simulink model "motorai"  (R2018b)
settings: Solver=FixedStepAuto  StartTime=0.0  StopTime=inf  FixedStep=SAMPLE_TIME  RelTol=1e-3
PreLoadFcn:
  | UserSettings
InitFcn:
  | ESTIMATION_SAMPLES = 50;
values from neighbouring files (symbols this model uses):
  ADC_bits = 12    [LQR_control_design.m]    (also in UserSettings.m)
  ADC_Vref = 3.3    [LQR_control_design.m]    (also in UserSettings.m)
  current_gain = 0.5    [LQR_control_design.m]    (also in UserSettings.m)
  current_offset = 1    [LQR_control_design.m]    (also in UserSettings.m)
  DATA_SAMPLING_FREQUENCY = 500    [UserSettings.m]
  K = -K    (= -0.383)    [LQG_control_design.m]    (also in LQR_control_design.m = -(1/R).*B'*Sinf; myLQR.m = -(1/R).*B'*Sinf; myREF.m = [Kw Ki])
  motorParameters = Parameters()    [UserSettings.m]
  omega_gain = 0.5    [LQR_control_design.m]    (also in UserSettings.m)
  omega_offset = 1    [LQR_control_design.m]    (also in UserSettings.m)
  PPR = 1000    [LQR_control_design.m]    (also in UserSettings.m)
  Q = 1/2*inv([(omega_max)^2 0 0; 0 (i_max)^2 0; 0 0 (int_max)^2])    [LQG_control_design.m]    (also in LQR_control_design.m = 1/2*inv([(omega_max)^2 0 ; 0 (i_max)^2]); myLQR.m = 1/2*inv([(omega_max)^2 0; 0 (i_max)^2]))
  R = inv([(v_max)^2])    [LQG_control_design.m]    (also in LQR_control_design.m; myLQR.m)
  SAMPLE_TIME = 5e-5    (= 5e-05)    [UserSettings.m]
  V_ACT = 12    [UserSettings.m]
  Vact = 12    [LQR_control_design.m]
undefined symbols (not defined in the file or in its folder): DiscIntNeverNeededParam
libraries: neural x275, mbedblockslib x7, fl_lib x5, nesl_utility x5, dspswit3 x3, elec_lib x3, powerlib_meascontrol x3, dspbuff3 x2, discretizing x1
(part 1 of 14)
settings Model: Creator=aaronrusso  LastModifiedBy=angel
settings DebuggingCC: LibraryContextMissingDiagnostic=none
settings SFSimCC: SimUseLocalCustomCode=off
settings RTWCC: RTWUseLocalCustomCode=off

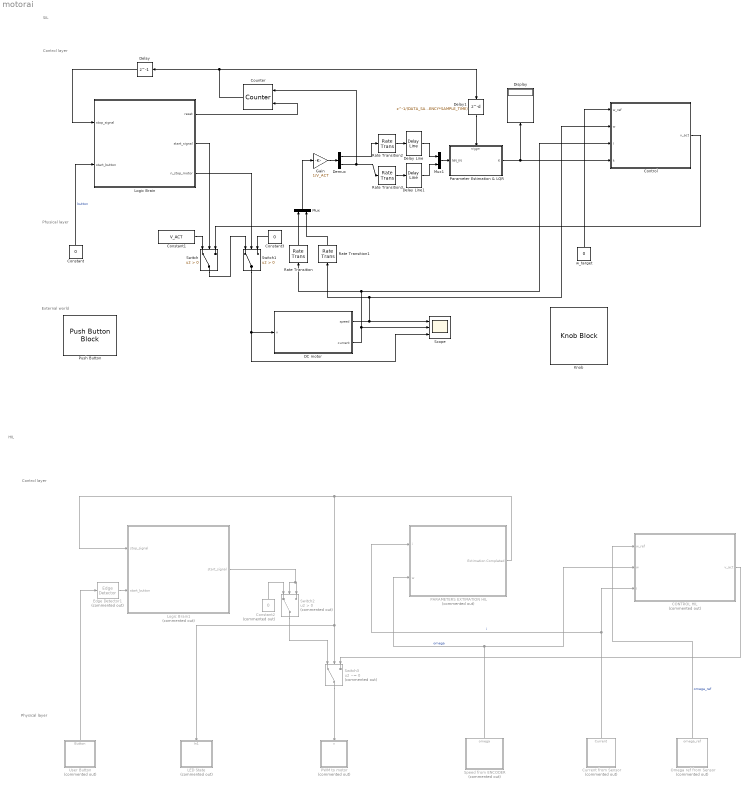
== system motorai ==
  note: HIL
  note: Control layer
  note: Physical layer
  note: External world
  note: Control layer
  note: Physical layer
  note: SIL
  CONTROL HIL : Subsystem  Commented=on
  Constant : Constant  Value=0  SampleTime=SAMPLE_TIME
  Constant1 : Constant  Value=V_ACT  SampleTime=SAMPLE_TIME
  Constant2 : Constant  Commented=on  Value=0
  Constant3 : Constant  Value=0
  "Control " : Subsystem  TreatAsAtomicUnit=on
  Counter : dspswit3/Counter  Direction=Up  CountEvent=Non-zero sample  CounterSize=User defined  MaxCount=(ESTIMATION_SAMPLES)/(DATA_SAMPLING_FREQUENCY*SAMPLE_TIME)  InitialCount=0  Output=Hit  HitValue=(ESTIMATION_SAMPLES)/(DATA_SAMPLING_FREQUENCY*SAMPLE_TIME)  ResetInput=on  SamplesPerFrame=1  Ts=1  CntDtype=double  HitDtype=Logical
  Current from Sensor : Subsystem  Commented=on
      mask Display: image('E:\Università\Magistrale - Advanced Automotive Electronic Engineering\Compliance Design of Automotive Systems\motor-control\MATLAB\images\lowres-INFIN_Icon_Current_02.eps.png');
  DC motor : Subsystem  ClipboardFcn=run('init_throttle.m')
  Delay : Delay  DelayLength=1  InitialCondition=0
  Delay Line : dspbuff3/Delay Line  siz=50  ic=0  directfeed=off  enable_output=off  hold_output=off  OutputFrames=off
      settings: SourceProductName=DSP System Toolbox  SourceProductBaseCode=DS
  Delay Line1 : dspbuff3/Delay Line  siz=50  ic=0  directfeed=off  enable_output=off  hold_output=off  OutputFrames=off
      settings: SourceProductName=DSP System Toolbox  SourceProductBaseCode=DS
  Delay1 : Delay  DelayLength=1/(DATA_SAMPLING_FREQUENCY*SAMPLE_TIME)  InitialCondition=0
  Demux : Demux  Outputs=2
  Display : Display
  Edge Detector1 : powerlib_meascontrol/Logic/Edge Detector  Commented=on  model=Rising  ic=0  Ts=0
      settings: SourceProductName=Simscape Power Systems  SourceProductBaseCode=PS
  Gain : Gain  Gain=1/V_ACT
  Knob : KnobBlock  WebBlockId=276  ScaleMax=500
  LED State : Subsystem  Commented=on
      mask Display: image('E:\Università\Magistrale - Advanced Automotive Electronic Engineering\Compliance Design of Automotive Systems\motor-control\MATLAB\images\led.png');
  Logic Brain : Stateflow chart  TreatAsAtomicUnit=on
  Logic Brain1 : Stateflow chart  Commented=on  TreatAsAtomicUnit=on
  Mux : Mux  Inputs=2
  Mux1 : Mux  Inputs=2
  Omega ref from Sensor : Subsystem  Commented=on
      mask Display: image('E:\Università\Magistrale - Advanced Automotive Electronic Engineering\Compliance Design of Automotive Systems\motor-control\MATLAB\images\65193.png');
  PARAMETERS EXTIMATION HIL : Subsystem  Commented=on
  PWM to motor : Subsystem  Commented=on
      mask Display: image('E:\Università\Magistrale - Advanced Automotive Electronic Engineering\Compliance Design of Automotive Systems\motor-control\MATLAB\images\PWM-Icon.png');
  "Parameter Estimation & LQR " : Subsystem  TreatAsAtomicUnit=on
  Push Button : PushButtonBlock  WebBlockId=163  LabelPosition=Top
  Rate Transition{,1..3} (4 alike) : RateTransition  OutPortSampleTime=1/DATA_SAMPLING_FREQUENCY
  Scope : Scope  NumInputPorts=3
  Speed from ENCODER : Subsystem  Commented=on
      mask Display: image('E:\Università\Magistrale - Advanced Automotive Electronic Engineering\Compliance Design of Automotive Systems\motor-control\MATLAB\images\Cattura.JPG');
  Switch : Switch  Criteria=u2 > Threshold
  Switch1 : Switch  Criteria=u2 > Threshold
  Switch2 : Switch  Commented=on  Criteria=u2 > Threshold
  Switch3 : Switch  Commented=on  Criteria=u2 ~= 0
  User Button : Subsystem  Commented=on
      mask Display: image('E:\Università\Magistrale - Advanced Automotive Electronic Engineering\Compliance Design of Automotive Systems\motor-control\MATLAB\images\red-start-button-5a28dc2fca5281.8598306415126272478287.jpg');
  w_target : Constant  Value=0
  wires:
  Logic Brain1/1(start_signal) -> Switch2/2, Switch2/3
  PARAMETERS EXTIMATION HIL/1(Extimation Completed) -> Logic Brain1/1(stop_signal), LED State/1(In1), Switch3/2
  Constant2/1 -> Switch2/1
  Edge Detector1/1 -> Logic Brain1/2(start_button)
  Current from Sensor/1(Current) -> CONTROL HIL/3(I), PARAMETERS EXTIMATION HIL/1(i)  "i"
  Speed from ENCODER/1(omega) -> CONTROL HIL/2(w), PARAMETERS EXTIMATION HIL/2(w)  "omega"
  Omega ref from Sensor/1(omega_ref) -> CONTROL HIL/1(w_ref)  "omega_ref"
  Switch2/1 -> Switch3/1
  CONTROL HIL/1(v_act) -> Switch3/3
  Switch3/1 -> PWM to motor/1(v)
  User Button/1(Button) -> Edge Detector1/1
  "Parameter Estimation & LQR "/1(K) -> "Control "/4(k), Display/1
  Demux/1 -> Rate Transition2/1
  Counter/1 -> Delay1/1, Delay/1
  Gain/1 -> Demux/1
  Rate Transition2/1 -> Delay Line/1
  Delay/1 -> Logic Brain/1(stop_signal)
  Rate Transition3/1 -> Delay Line1/1
  Rate Transition/1 -> Mux/1
  Rate Transition1/1 -> Mux/2
  Delay Line/1 -> Mux1/1
  Demux/2 -> Rate Transition3/1, Counter/1
  Delay Line1/1 -> Mux1/2
  Delay1/1 -> "Parameter Estimation & LQR "/Trigger
  Mux/1 -> Gain/1
  Mux1/1 -> "Parameter Estimation & LQR "/1(NN_IN)
  Constant/1 -> Logic Brain/2(start_button)  "button"
  Logic Brain/1(reset) -> Counter/2
  Logic Brain/2(start_signal) -> Switch/2
  DC motor/1(speed) -> Scope/1, "Control "/2(w), Rate Transition1/1
  Constant1/1 -> Switch/1
  "Control "/1(v_act) -> Switch/3
  w_target/1 -> "Control "/1(w_ref)
  DC motor/2(current) -> Scope/2, "Control "/3(I), Rate Transition/1
  Logic Brain/3(n_stop_motor) -> Switch1/2
  Switch/1 -> Switch1/1
  Constant3/1 -> Switch1/3
  Switch1/1 -> Scope/3, DC motor/1(v)

== system motorai/CONTROL HIL ==
  w_ref : Inport
  w : Inport  Port=2
  I : Inport  Port=3
  LQR control sim : Subsystem
  Mux1 : Mux  Inputs=2
  v_act : Outport
  wires:
  LQR control sim/1(u) -> v_act/1
  w_ref/1 -> LQR control sim/2(y_ref)
  w/1 -> Mux1/1
  I/1 -> Mux1/2
  Mux1/1 -> LQR control sim/1(x)

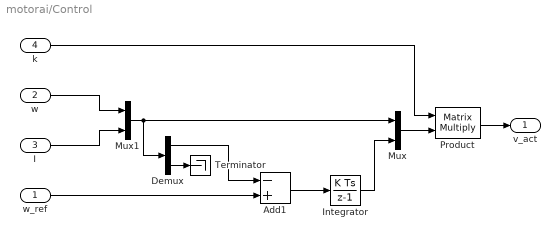
== system motorai/Control  ==
  w_ref : Inport
  w : Inport  Port=2
  I : Inport  Port=3
  k : Inport  Port=4
  Add1 : Sum  Inputs=-+
  Demux : Demux  Outputs=2
  Integrator : DiscreteIntegrator  SampleTime=1.0  ICPrevOutput=DiscIntNeverNeededParam  ICPrevScaledInput=DiscIntNeverNeededParam  mask(DiscretizedDiscreteIntegrator){}
      mask init:
      | %zoh
  Mux : Mux  Inputs=2
  Mux1 : Mux  Inputs=2
  Product : Product  Multiplication=Matrix(*)
  Terminator : Terminator
  v_act : Outport
  wires:
  Integrator/1 -> Mux/2
  Demux/1 -> Add1/1
  I/1 -> Mux1/2
  Product/1 -> v_act/1
  Demux/2 -> Terminator/1
  Add1/1 -> Integrator/1
  w/1 -> Mux1/1
  Mux1/1 -> Mux/1, Demux/1
  w_ref/1 -> Add1/2
  Mux/1 -> Product/2
  k/1 -> Product/1

== system motorai/Current from Sensor ==
  Add : Sum
  Analog Input : mbedblockslib/Analog Input  Pin=PB_0  ReadResultsOnly=off  ConversionTriggerSource=Software  ExternalTriggerType=uint32( 0 )  OutputDataType=double  EnableConversionCompleteNotify=off  EnableOuputStatus=off  SampleTime=-1
      settings: SourceProductName=Simulink Coder Support Package for BBC microbit Board  SourceProductBaseCode=MICROBIT
  current_gain : Gain  Gain=current_gain
  current_offset : Constant  Value=current_offset
  to Volts : Gain  Gain=ADC_Vref/(2^ADC_bits)
  Current : Outport
  wires:
  Analog Input/1 -> to Volts/1  "word"
  current_gain/1 -> Add/1
  current_offset/1 -> Add/2
  to Volts/1 -> current_gain/1  "volts"
  Add/1 -> Current/1  "Ampere"

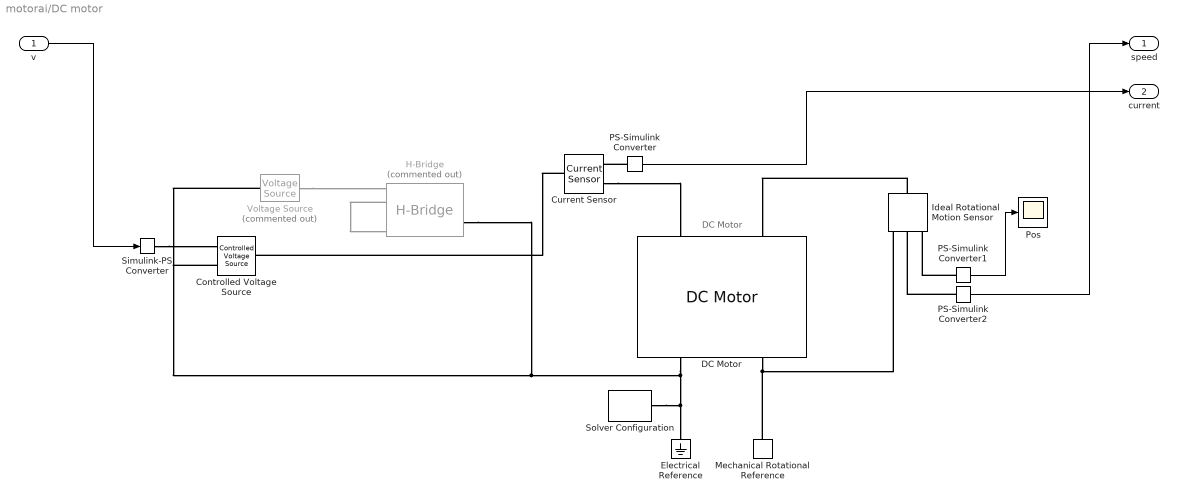
== system motorai/DC motor ==
  note: DC Motor
  v : Inport
  Controlled Voltage Source : fl_lib/Electrical/Electrical Sources/Controlled Voltage Source
  Current Sensor : fl_lib/Electrical/Electrical Sensors/Current Sensor
  DC Motor : elec_lib/Actuators & Drivers/Rotational Actuators/DC Motor  parameterization=1  Ra=1.15 Ohm  La=1.5 mH  emf_or_torque=1  Kv=0.383 V/(rad/s)  Ki=6.876e-4 N*m/A  T_stall=0.24e-3 N*m  w_max=19100 rpm  w_rated=15000 rpm  P_rated=0.08 W  V_rated=1.5 V  J=0.021 kg*m^2  lam_param=1  lam=0.087 N*m/(rad/s)  i_noload=0 A  V_i_noload=1.5 V  speed0=10 rad/s  alpha=3.93e-3 1/K  Tmeas=25 degC  thermal_mass=100 J/K  initial_temperature=25 degC
  Electrical Reference : fl_lib/Electrical/Electrical Elements/Electrical Reference
  H-Bridge : elec_lib/Actuators & Drivers/Drivers/H-Bridge  Commented=on  Venable=2.5 V  Vmax=5.0 V  Vreverse=2.5 V  Vbrake=2.5 V  Vm=12 V  pwm_or_av=1  discontinuous=0  freewheeling_mode=1  freewheeling_mode_disc=1  Ron=0.1 Ohm  Don=0.05 Ohm  Rload=10 Ohm  Lload=1e-5 H  F=10 kHz  thermal_mass=100 J/K  initial_temperature=298.15 K  Ron2=0.1 Ohm  Don2=0.05 Ohm  Tmeas=298.15 K  Tmeas2=398.15 K
      settings: SourceProductName=Simscape Electronics  SourceProductBaseCode=SN
  Ideal Rotational Motion Sensor : fl_lib/Mechanical/Mechanical Sensors/Ideal Rotational Motion Sensor  offset=0 rad
  Mechanical Rotational Reference : fl_lib/Mechanical/Rotational Elements/Mechanical Rotational Reference
  PS-Simulink Converter : nesl_utility/PS-Simulink Converter  PhysicalDomain=network_engine_domain  SubClassName=ps_output  LeftPortType=input  RightPortType=output  PseudoPeriodic=off  Frequencies=[]  Unit=A  AffineConversion=off
  PS-Simulink Converter1 : nesl_utility/PS-Simulink Converter  PhysicalDomain=network_engine_domain  SubClassName=ps_output  LeftPortType=input  RightPortType=output  PseudoPeriodic=off  Frequencies=[]  Unit=rad  AffineConversion=off
  PS-Simulink Converter2 : nesl_utility/PS-Simulink Converter  PhysicalDomain=network_engine_domain  SubClassName=ps_output  LeftPortType=input  RightPortType=output  PseudoPeriodic=off  Frequencies=[]  Unit=rad/s  AffineConversion=off
  Pos : Scope
  Simulink-PS Converter : nesl_utility/Simulink-PS Converter  PhysicalDomain=network_engine_domain  SubClassName=ps_input  LeftPortType=input  RightPortType=output  PseudoPeriodic=off  Frequencies=[]  NoiseDistribution=none  NoiseParameters=[]  Unit=V  AffineConversion=off  FilteringAndDerivatives=provide  SimscapeFilterOrder=1  InputFilterTimeConstant=0.001  UdotUserProvided=0
  Solver Configuration : nesl_utility/Solver Configuration  PhysicalDomain=network_engine_domain  SubClassName=solver  LeftPortType=input  RightPortType=generic  Tones=[]  Harmonics=[]  SimulateNoise=off  Profile=off  UseLocalSampling=off  EnableSwitchedLinearOptims=on  FrequencyDomain=off  UseCCode=off  RelTol=0.001  AbsTol=1e-06  MinStep=1e-09  ToWorkspace=off  RevertToSquareIcSolve=off  NumHomotopyIterations=100  PhasorMode=off  PhasorModeNumHarmonics=1  DoDC=off  ResidualTolerance=1e-09  UseLocalSolver=off  LocalSolverChoice=NE_BACKWARD_EULER_ADVANCER  LocalSolverSampleTime=0.001  DoFixedCost=off  MaxNonlinIter=3  MaxModeIter=2  LinearAlgebra=auto  EquationFormulation=NE_TIME_EF  DelaysMemoryBudget=1024  AutomaticFiltering=on  FilteringTimeConstant=0.001  PartitionStorageMethod=AS_NEEDED  PartitionMemoryBudget=1024
  Voltage Source : elec_lib/Sources/Voltage Source  Commented=on  dc_voltage=12 V  ac_voltage=0 V  ac_shift=0 rad  ac_frequency=60 Hz  noise_mode=0  PSD=0 V^2/Hz  repeatability=1  auto_seed=3890346746  user_seed=0  sample_time=1e-3 s  i_specify=off  i_priority=None  i=0 A  i_nominal_specify=off  i_nominal_unit=A  i_nominal_value=1  v_specify=off  v_priority=None  v=0 V  v_nominal_specify=off  v_nominal_unit=V  v_nominal_value=1
      settings: SourceProductName=Simscape Electronics  SourceProductBaseCode=SN
  speed : Outport
  current : Outport  Port=2
  wires:
  PS-Simulink Converter2/1 -> speed/1
  v/1 -> Simulink-PS Converter/1
  PS-Simulink Converter1/1 -> Pos/1
  PS-Simulink Converter/1 -> current/1
  connections:
  Ideal Rotational Motion Sensor/LConn1 -- DC Motor/LConn2
  DC Motor/RConn2 -- Ideal Rotational Motion Sensor/RConn1 -- Mechanical Rotational Reference/LConn1
  DC Motor/RConn1 -- Voltage Source/RConn1 -- Controlled Voltage Source/RConn2 -- H-Bridge/RConn2 -- Solver Configuration/RConn1 -- Electrical Reference/LConn1
  Current Sensor/RConn2 -- DC Motor/LConn1
  PS-Simulink Converter/LConn1 -- Current Sensor/RConn1
  Simulink-PS Converter/RConn1 -- Controlled Voltage Source/RConn1
  Voltage Source/LConn1 -- H-Bridge/LConn1
  PS-Simulink Converter1/LConn1 -- Ideal Rotational Motion Sensor/RConn3
  PS-Simulink Converter2/LConn1 -- Ideal Rotational Motion Sensor/RConn2
  Current Sensor/LConn1 -- Controlled Voltage Source/LConn1
  H-Bridge/LConn2 -- H-Bridge/LConn4

== system motorai/LED State ==
  In1 : Inport
  Digital Write : mbedblockslib/Digital Write  Pin=PA_5  Direction=output
      settings: SourceProductName=Simulink Coder Support Package for BBC microbit Board  SourceProductBaseCode=MICROBIT
  NOT : Logic  Operator=NOT  IconShape=distinctive  AllPortsSameDT=off  OutDataTypeStr=boolean
  wires:
  In1/1 -> NOT/1
  NOT/1 -> Digital Write/1

== system motorai/Omega ref from Sensor ==
  Add : Sum
  Analog Input : mbedblockslib/Analog Input  Pin=PC_0  ReadResultsOnly=off  ConversionTriggerSource=Software  ExternalTriggerType=uint32( 0 )  OutputDataType=double  EnableConversionCompleteNotify=off  EnableOuputStatus=off  SampleTime=-1
      settings: SourceProductName=Simulink Coder Support Package for BBC microbit Board  SourceProductBaseCode=MICROBIT
  omega_gain : Gain  Gain=omega_gain
  omega_offset : Constant  Value=omega_offset
  to Volts : Gain  Gain=ADC_Vref/(2^ADC_bits)
  omega_ref : Outport
  wires:
  Add/1 -> omega_ref/1  "rad/s"
  to Volts/1 -> omega_gain/1  "volts"
  omega_offset/1 -> Add/2
  omega_gain/1 -> Add/1
  Analog Input/1 -> to Volts/1  "word"

== system motorai/PARAMETERS EXTIMATION HIL ==
  i : Inport
  w : Inport  Port=2
  Edge Detector : dspswit3/Edge Detector  InputProcessing=Columns as channels (frame based)
      settings: SourceProductName=DSP System Toolbox  SourceProductBaseCode=DS
  Function Fitting Neural Network : Subsystem
      mask help: Function Fitting Neural Network
      mask Display: e = 0.06;c1 = [120 150 230]/255;c2 = ([120 150 230]+0)/383;c3 = ([120 150 230]+128)/383;patch([0 1 1 0],[0 0 1 1],c1);patch([0 1 1 1-e 1-e 0+e],[0 0 1 1-e 0+e 0+e],c2);patch([0 0 1 1-e 0+e 0+e],[0 1 1 1-e 1-e 0+e],c3);plot([0 1 1 0 0],[0 0 1 1 0]);fprintf('NNET');port_label('input',1,' Input');port_label('output',1,'Output ');
  Vector Concatenate : Concatenate
  i_buffer : Buffer  N=ESTIMATION_SAMPLES  OutputFrames=off
  w_buffer1 : Buffer  N=ESTIMATION_SAMPLES  OutputFrames=off
  y1 : Scope
      mask Display: e = 0.06;c1 = [120 230 180]/255;c2 = ([120 230 180]+0)/(256+128);c3 = ([120 230 180]+128)/(256+128);patch([0 1 1 0],[0 0 1 1],c1);patch([0 1 1 1-e 1-e 0+e],[0 0 1 1-e 0+e 0+e],c2);patch([0 0 1 1-e 0+e 0+e],[0 1 1 1-e 1-e 0+e],c3);plot([0 1 1 0 0],[0 0 1 1 0]);plot([0.15 0.85 0.85 0.15 0.15],[0.5 0.5 0.85 0.85 0.5]);
  Extimation Completed : Outport
  wires:
  Function Fitting Neural Network/1(Output) -> y1/1
  w/1 -> w_buffer1/1
  Vector Concatenate/1 -> Edge Detector/1, Function Fitting Neural Network/1(Input)
  Edge Detector/1 -> Extimation Completed/1
  w_buffer1/1 -> Vector Concatenate/2
  i_buffer/1 -> Vector Concatenate/1
  i/1 -> i_buffer/1

== system motorai/PWM to motor ==
  v : Inport
  Actuation voltage : Constant  Value=Vact
  Divide : Product  Inputs=*/
  Divide1 : Product  Inputs=**
  PWM Output : mbedblockslib/PWM Output  Pin=PA_3  EnableInputFrequency=off  InitialFrequency=2000  InitialDutyCycle=50  NotificationType=None
      settings: SourceProductName=Simulink Coder Support Package for BBC microbit Board  SourceProductBaseCode=MICROBIT
  to percentage : Constant  Value=100
  wires:
  Actuation voltage/1 -> Divide/2
  v/1 -> Divide/1
  Divide/1 -> Divide1/1
  to percentage/1 -> Divide1/2
  Divide1/1 -> PWM Output/1

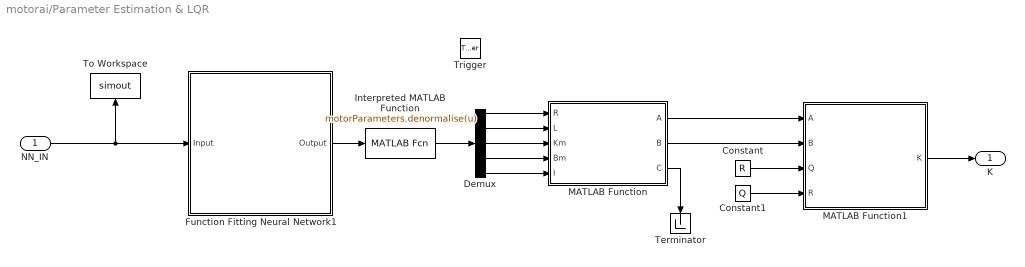
== system motorai/Parameter Estimation & LQR  ==
  NN_IN : Inport
  Trigger : TriggerPort  VariantControl=Variant
  Constant : Constant  Value=R
  Constant1 : Constant  Value=Q
  Demux : Demux  Outputs=5
  Function Fitting Neural Network1 : Subsystem
      mask help: Function Fitting Neural Network
      mask Display: e = 0.06;c1 = [120 150 230]/255;c2 = ([120 150 230]+0)/383;c3 = ([120 150 230]+128)/383;patch([0 1 1 0],[0 0 1 1],c1);patch([0 1 1 1-e 1-e 0+e],[0 0 1 1-e 0+e 0+e],c2);patch([0 0 1 1-e 0+e 0+e],[0 1 1 1-e 1-e 0+e],c3);plot([0 1 1 0 0],[0 0 1 1 0]);fprintf('NNET');port_label('input',1,' Input');port_label('output',1,'Output ');
  Interpreted MATLAB Function : MATLABFcn  MATLABFcn=motorParameters.denormalise(u)
  MATLAB Function : MATLAB Function  TreatAsAtomicUnit=on
  MATLAB Function1 : MATLAB Function  TreatAsAtomicUnit=on
  Terminator : Terminator
  To Workspace : ToWorkspace  VariableName=simout  SaveFormat=Timeseries  SampleTime=-1
  K : Outport
  wires:
  Function Fitting Neural Network1/1(Output) -> Interpreted MATLAB Function/1
  NN_IN/1 -> Function Fitting Neural Network1/1(Input), To Workspace/1
  Interpreted MATLAB Function/1 -> Demux/1
  Demux/1 -> MATLAB Function/1(R)
  Demux/2 -> MATLAB Function/2(L)
  Demux/3 -> MATLAB Function/3(Km)
  Demux/4 -> MATLAB Function/4(Bm)
  Demux/5 -> MATLAB Function/5(I)
  MATLAB Function/3(C) -> Terminator/1
  MATLAB Function/1(A) -> MATLAB Function1/1(A)
  MATLAB Function/2(B) -> MATLAB Function1/2(B)
  Constant/1 -> MATLAB Function1/3(Q)
  Constant1/1 -> MATLAB Function1/4(R)
  MATLAB Function1/1(K) -> K/1

== system motorai/Speed from ENCODER ==
  note: ONLY ONE DIRECTION
      | needs work
  Counter : dspswit3/Counter  Direction=Up  CountEvent=Rising edge  CounterSize=User defined  MaxCount=255  InitialCount=0  Output=Count and Hit  HitValue=32  ResetInput=off  SamplesPerFrame=1  Ts=1  CntDtype=double  HitDtype=Logical
  Derivative : discretizing/Discretized Derivative  method=tustin  SampleTime=1.0  Wc=1
  ENC_A : mbedblockslib/Digital Read  Pin=PA_0  Direction=input  SampleTime=-1
      settings: SourceProductName=Simulink Coder Support Package for BBC microbit Board  SourceProductBaseCode=MICROBIT
  ENC_B : mbedblockslib/Digital Read  Pin=PA_1  Direction=input  SampleTime=-1
      settings: SourceProductName=Simulink Coder Support Package for BBC microbit Board  SourceProductBaseCode=MICROBIT
  Gain : Gain  Gain=2*pi/PPR
  Quadrature Decoder : Subsystem
  Terminator : Terminator
  omega : Outport
  wires:
  ENC_A/1 -> Quadrature Decoder/1(A)
  ENC_B/1 -> Quadrature Decoder/2(B)
  Quadrature Decoder/2(COUNT) -> Counter/1
  Counter/1 -> Gain/1  "#pulses"
  Gain/1 -> Derivative/1  "rad"
  Derivative/1 -> omega/1  "rad/s"
  Counter/2 -> Terminator/1

== system motorai/User Button ==
  Digital Read : mbedblockslib/Digital Read  Pin=PC_13  Direction=input  SampleTime=-1
      settings: SourceProductName=Simulink Coder Support Package for BBC microbit Board  SourceProductBaseCode=MICROBIT
  Button : Outport
  wires:
  Digital Read/1 -> Button/1

== system motorai/CONTROL HIL/LQR control sim ==
  x : Inport
  y_ref : Inport  Port=2
  Add1 : Sum  Inputs=-+
  Demux : Demux  Outputs=2
  Gain : Gain  Gain=K  Multiplication=Matrix(K*u) (u vector)
  Integrator : DiscreteIntegrator  SampleTime=1.0  ICPrevOutput=DiscIntNeverNeededParam  ICPrevScaledInput=DiscIntNeverNeededParam  mask(DiscretizedDiscreteIntegrator){}
      mask init:
      | %zoh
  Mux : Mux  Inputs=2
  Terminator : Terminator
  u : Outport
  wires:
  Mux/1 -> Gain/1
  Demux/1 -> Add1/1
  y_ref/1 -> Add1/2
  Gain/1 -> u/1
  Integrator/1 -> Mux/2
  Add1/1 -> Integrator/1
  x/1 -> Mux/1, Demux/1
  Demux/2 -> Terminator/1

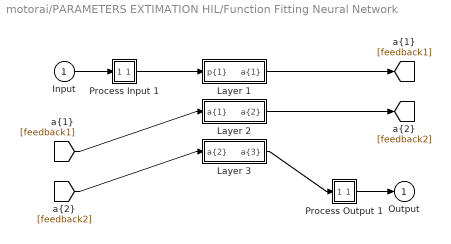
== system motorai/PARAMETERS EXTIMATION HIL/Function Fitting Neural Network ==
  Input : Inport  PortDimensions=100
      mask Display: e = 0.06;c1 = [120 230 180]/255;c2 = ([120 230 180]+0)/(256+128);c3 = ([120 230 180]+128)/(256+128);patch([0 1 1 0],[0 0 1 1],c1);patch([0 1 1 1-e 1-e 0+e],[0 0 1 1-e 0+e 0+e],c2);patch([0 0 1 1-e 0+e 0+e],[0 1 1 1-e 1-e 0+e],c3);plot([0 1 1 0 0],[0 0 1 1 0]);
  Layer 1 : Subsystem
      mask Display: e = 0.06;c1 = [120 150 230]/255;c2 = ([120 150 230]+0)/383;c3 = ([120 150 230]+128)/383;patch([0 1 1 0],[0 0 1 1],c1);patch([0 1 1 1-e 1-e 0+e],[0 0 1 1-e 0+e 0+e],c2);patch([0 0 1 1-e 0+e 0+e],[0 1 1 1-e 1-e 0+e],c3);plot([0 1 1 0 0],[0 0 1 1 0]);
  Layer 2 : Subsystem
      mask Display: e = 0.06;c1 = [120 150 230]/255;c2 = ([120 150 230]+0)/383;c3 = ([120 150 230]+128)/383;patch([0 1 1 0],[0 0 1 1],c1);patch([0 1 1 1-e 1-e 0+e],[0 0 1 1-e 0+e 0+e],c2);patch([0 0 1 1-e 0+e 0+e],[0 1 1 1-e 1-e 0+e],c3);plot([0 1 1 0 0],[0 0 1 1 0]);
  Layer 3 : Subsystem
      mask Display: e = 0.06;c1 = [120 150 230]/255;c2 = ([120 150 230]+0)/383;c3 = ([120 150 230]+128)/383;patch([0 1 1 0],[0 0 1 1],c1);patch([0 1 1 1-e 1-e 0+e],[0 0 1 1-e 0+e 0+e],c2);patch([0 0 1 1-e 0+e 0+e],[0 1 1 1-e 1-e 0+e],c3);plot([0 1 1 0 0],[0 0 1 1 0]);
  Process Input 1 : Subsystem
      mask Display: e = 0.06;c1 = [120 150 230]/255;c2 = ([120 150 230]+0)/383;c3 = ([120 150 230]+128)/383;patch([0 1 1 0],[0 0 1 1],c1);patch([0 1 1 1-e 1-e 0+e],[0 0 1 1-e 0+e 0+e],c2);patch([0 0 1 1-e 0+e 0+e],[0 1 1 1-e 1-e 0+e],c3);plot([0 1 1 0 0],[0 0 1 1 0]);
  Process Output 1 : Subsystem
      mask Display: e = 0.06;c1 = [120 150 230]/255;c2 = ([120 150 230]+0)/383;c3 = ([120 150 230]+128)/383;patch([0 1 1 0],[0 0 1 1],c1);patch([0 1 1 1-e 1-e 0+e],[0 0 1 1-e 0+e 0+e],c2);patch([0 0 1 1-e 0+e 0+e],[0 1 1 1-e 1-e 0+e],c3);plot([0 1 1 0 0],[0 0 1 1 0]);
  Output : Outport  InitialOutput=[0;0;0;0;0]
      mask Display: e = 0.06;c1 = [120 230 180]/255;c2 = ([120 230 180]+0)/(256+128);c3 = ([120 230 180]+128)/(256+128);patch([0 1 1 0],[0 0 1 1],c1);patch([0 1 1 1-e 1-e 0+e],[0 0 1 1-e 0+e 0+e],c2);patch([0 0 1 1-e 0+e 0+e],[0 1 1 1-e 1-e 0+e],c3);plot([0 1 1 0 0],[0 0 1 1 0]);
  wires:
  Layer 3/1("a{3}") -> Process Output 1/1(a)
  [feedback2] -> Layer 3/1("a{2} ")
  Layer 2/1("a{2}") -> [feedback2]
  [feedback1] -> Layer 2/1("a{1} ")
  Layer 1/1("a{1}") -> [feedback1]
  Process Input 1/1(p) -> Layer 1/1("p{1}")
  Process Output 1/1(y) -> Output/1
  Input/1 -> Process Input 1/1(x)

== system motorai/Parameter Estimation & LQR /Function Fitting Neural Network1 ==
  Input : Inport  PortDimensions=100
      mask Display: e = 0.06;c1 = [120 230 180]/255;c2 = ([120 230 180]+0)/(256+128);c3 = ([120 230 180]+128)/(256+128);patch([0 1 1 0],[0 0 1 1],c1);patch([0 1 1 1-e 1-e 0+e],[0 0 1 1-e 0+e 0+e],c2);patch([0 0 1 1-e 0+e 0+e],[0 1 1 1-e 1-e 0+e],c3);plot([0 1 1 0 0],[0 0 1 1 0]);
  Layer 1 : Subsystem
      mask Display: e = 0.06;c1 = [120 150 230]/255;c2 = ([120 150 230]+0)/383;c3 = ([120 150 230]+128)/383;patch([0 1 1 0],[0 0 1 1],c1);patch([0 1 1 1-e 1-e 0+e],[0 0 1 1-e 0+e 0+e],c2);patch([0 0 1 1-e 0+e 0+e],[0 1 1 1-e 1-e 0+e],c3);plot([0 1 1 0 0],[0 0 1 1 0]);
  Layer 2 : Subsystem
      mask Display: e = 0.06;c1 = [120 150 230]/255;c2 = ([120 150 230]+0)/383;c3 = ([120 150 230]+128)/383;patch([0 1 1 0],[0 0 1 1],c1);patch([0 1 1 1-e 1-e 0+e],[0 0 1 1-e 0+e 0+e],c2);patch([0 0 1 1-e 0+e 0+e],[0 1 1 1-e 1-e 0+e],c3);plot([0 1 1 0 0],[0 0 1 1 0]);
  Layer 3 : Subsystem
      mask Display: e = 0.06;c1 = [120 150 230]/255;c2 = ([120 150 230]+0)/383;c3 = ([120 150 230]+128)/383;patch([0 1 1 0],[0 0 1 1],c1);patch([0 1 1 1-e 1-e 0+e],[0 0 1 1-e 0+e 0+e],c2);patch([0 0 1 1-e 0+e 0+e],[0 1 1 1-e 1-e 0+e],c3);plot([0 1 1 0 0],[0 0 1 1 0]);
  Process Input 1 : Subsystem
      mask Display: e = 0.06;c1 = [120 150 230]/255;c2 = ([120 150 230]+0)/383;c3 = ([120 150 230]+128)/383;patch([0 1 1 0],[0 0 1 1],c1);patch([0 1 1 1-e 1-e 0+e],[0 0 1 1-e 0+e 0+e],c2);patch([0 0 1 1-e 0+e 0+e],[0 1 1 1-e 1-e 0+e],c3);plot([0 1 1 0 0],[0 0 1 1 0]);
  Process Output 1 : Subsystem
      mask Display: e = 0.06;c1 = [120 150 230]/255;c2 = ([120 150 230]+0)/383;c3 = ([120 150 230]+128)/383;patch([0 1 1 0],[0 0 1 1],c1);patch([0 1 1 1-e 1-e 0+e],[0 0 1 1-e 0+e 0+e],c2);patch([0 0 1 1-e 0+e 0+e],[0 1 1 1-e 1-e 0+e],c3);plot([0 1 1 0 0],[0 0 1 1 0]);
  Output : Outport  InitialOutput=[0;0;0;0;0]
      mask Display: e = 0.06;c1 = [120 230 180]/255;c2 = ([120 230 180]+0)/(256+128);c3 = ([120 230 180]+128)/(256+128);patch([0 1 1 0],[0 0 1 1],c1);patch([0 1 1 1-e 1-e 0+e],[0 0 1 1-e 0+e 0+e],c2);patch([0 0 1 1-e 0+e 0+e],[0 1 1 1-e 1-e 0+e],c3);plot([0 1 1 0 0],[0 0 1 1 0]);
  wires:
  Input/1 -> Process Input 1/1(x)
  Process Output 1/1(y) -> Output/1
  Process Input 1/1(p) -> Layer 1/1("p{1}")
  Layer 1/1("a{1}") -> [feedback1]
  [feedback1] -> Layer 2/1("a{1} ")
  Layer 2/1("a{2}") -> [feedback2]
  [feedback2] -> Layer 3/1("a{2} ")
  Layer 3/1("a{3}") -> Process Output 1/1(a)

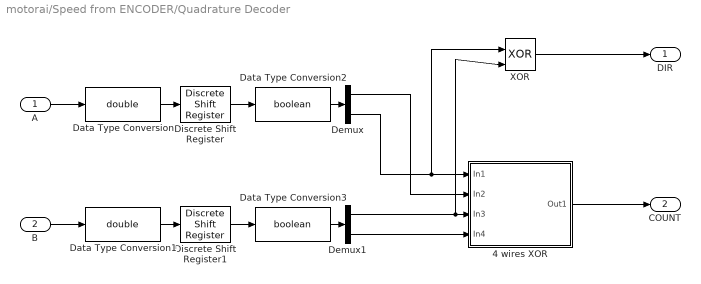
== system motorai/Speed from ENCODER/Quadrature Decoder ==
  A : Inport
  B : Inport  Port=2
  4 wires XOR : Subsystem
  Data Type Conversion : DataTypeConversion  OutDataTypeStr=double
  Data Type Conversion1 : DataTypeConversion  OutDataTypeStr=double
  Data Type Conversion2 : DataTypeConversion  OutDataTypeStr=boolean
  Data Type Conversion3 : DataTypeConversion  OutDataTypeStr=boolean
  Demux : Demux  Outputs=2
  Demux1 : Demux  Outputs=2
  Discrete Shift Register : powerlib_meascontrol/Additional Components/Discrete Shift Register  NSamples=2  InitialValue=0  Ts=50e-6
      settings: SourceProductName=Simscape Electrical  SourceProductBaseCode=PS
  Discrete Shift Register1 : powerlib_meascontrol/Additional Components/Discrete Shift Register  NSamples=2  InitialValue=0  Ts=50e-6
      settings: SourceProductName=Simscape Electrical  SourceProductBaseCode=PS
  XOR : Logic  Operator=XOR  IconShape=distinctive  AllPortsSameDT=off  OutDataTypeStr=boolean
  DIR : Outport
  COUNT : Outport  Port=2
  wires:
  4 wires XOR/1(Out1) -> COUNT/1
  Demux/1 -> 4 wires XOR/2(In2)
  Demux/2 -> XOR/1, 4 wires XOR/1(In1)
  Demux1/1 -> XOR/2, 4 wires XOR/3(In3)
  Demux1/2 -> 4 wires XOR/4(In4)
  XOR/1 -> DIR/1
  A/1 -> Data Type Conversion/1
  Data Type Conversion/1 -> Discrete Shift Register/1
  Data Type Conversion1/1 -> Discrete Shift Register1/1
  B/1 -> Data Type Conversion1/1
  Discrete Shift Register/1 -> Data Type Conversion2/1
  Data Type Conversion2/1 -> Demux/1
  Discrete Shift Register1/1 -> Data Type Conversion3/1
  Data Type Conversion3/1 -> Demux1/1

== system motorai/PARAMETERS EXTIMATION HIL/Function Fitting Neural Network/Layer 1 ==
  "p{1}" : Inport  PortDimensions=98
      mask Display: e = 0.06;c1 = [120 230 180]/255;c2 = ([120 230 180]+0)/(256+128);c3 = ([120 230 180]+128)/(256+128);patch([0 1 1 0],[0 0 1 1],c1);patch([0 1 1 1-e 1-e 0+e],[0 0 1 1-e 0+e 0+e],c2);patch([0 0 1 1-e 0+e 0+e],[0 1 1 1-e 1-e 0+e],c3);plot([0 1 1 0 0],[0 0 1 1 0]);
  Delays 1 : Subsystem
      mask Display: e = 0.06;c1 = [120 150 230]/255;c2 = ([120 150 230]+0)/383;c3 = ([120 150 230]+128)/383;patch([0 1 1 0],[0 0 1 1],c1);patch([0 1 1 1-e 1-e 0+e],[0 0 1 1-e 0+e 0+e],c2);patch([0 0 1 1-e 0+e 0+e],[0 1 1 1-e 1-e 0+e],c3);plot([0 1 1 0 0],[0 0 1 1 0]);disp('0');
  "IW{1,1}" : Subsystem
      mask Display: e = 0.06;c1 = [120 150 230]/255;c2 = ([120 150 230]+0)/383;c3 = ([120 150 230]+128)/383;patch([0 1 1 0],[0 0 1 1],c1);patch([0 1 1 1-e 1-e 0+e],[0 0 1 1-e 0+e 0+e],c2);patch([0 0 1 1-e 0+e 0+e],[0 1 1 1-e 1-e 0+e],c3);plot([0 1 1 0 0],[0 0 1 1 0]);disp('W');
  "b{1}" : Constant  Value=[-3.2035277209804444709106974187307059764862060546875;-25.49776091518986476103236782364547252655029296875;4.8692308933402816961688586161471903324127197265625;-2.9602967414270384693963933386839926242828369140625;-3.392277162648143384870991212665103375911712646484375;-1.6702173206823991424840869512991048395633697509765625;0.66445821251272840779478201511665247380733489990234375;5.3214322739079076285406699753366410732269287109375;9.3808541339032398553854363854043185710906982421875;1.7709888695075035602854995886445976793766021728515625;-2.97561860289332091866754126385785639286041259765625;5.37946098877317613329296364099718630313873291015625;1.0650209820557783313432764771278016269207000732421875;-0.4170133083953555530598578116041608154773712158203125;6.08009558138170991270499143865890800952911376953125;-9.7715355749550969477468242985196411609649658203125;-5.36036304535452590158683960908092558383941650390625;6.756780068120946225462830625474452972412109375;-7.90739342639891606978608251665718853473663330078125;4.3065835551293414340534582152031362056732177734375;-17.187268285240609344555196003057062625885009765625;-19.57276992687204852927607134915888309478759765625]
      mask Display: e = 0.06;c1 = [120 150 230]/255;c2 = ([120 150 230]+0)/383;c3 = ([120 150 230]+128)/383;patch([0 1 1 0],[0 0 1 1],c1);patch([0 1 1 1-e 1-e 0+e],[0 0 1 1-e 0+e 0+e],c2);patch([0 0 1 1-e 0+e 0+e],[0 1 1 1-e 1-e 0+e],c3);plot([0 1 1 0 0],[0 0 1 1 0]);disp('b');
  netsum : Sum  Inputs=2  SaturateOnIntegerOverflow=on  InputSameDT=on  OutDataTypeStr=Inherit: Same as first input
      mask Display: e = 0.06;c1 = [120 150 230]/255;c2 = ([120 150 230]+0)/383;c3 = ([120 150 230]+128)/383;patch([0 1 1 0],[0 0 1 1],c1);patch([0 1 1 1-e 1-e 0+e],[0 0 1 1-e 0+e 0+e],c2);patch([0 0 1 1-e 0+e 0+e],[0 1 1 1-e 1-e 0+e],c3);plot([0 1 1 0 0],[0 0 1 1 0]);disp('+');
  tansig : neural/Transfer Functions/tansig
      settings: SourceProductName=Deep Learning Toolbox
  "a{1}" : Outport  InitialOutput=[0;0;0;0;0;0;0;0;0;0;0;0;0;0;0;0;0;0;0;0;0;0]
      mask Display: e = 0.06;c1 = [120 230 180]/255;c2 = ([120 230 180]+0)/(256+128);c3 = ([120 230 180]+128)/(256+128);patch([0 1 1 0],[0 0 1 1],c1);patch([0 1 1 1-e 1-e 0+e],[0 0 1 1-e 0+e 0+e],c2);patch([0 0 1 1-e 0+e 0+e],[0 1 1 1-e 1-e 0+e],c3);plot([0 1 1 0 0],[0 0 1 1 0]);
  wires:
  tansig/1 -> "a{1}"/1
  netsum/1 -> tansig/1
  "b{1}"/1 -> netsum/2
  "IW{1,1}"/1("iz{1,1}") -> netsum/1
  Delays 1/1("pd{1,1}") -> "IW{1,1}"/1("pd{1,1}")
  "p{1}"/1 -> Delays 1/1("p{1}")

== system motorai/PARAMETERS EXTIMATION HIL/Function Fitting Neural Network/Layer 2 ==
  "a{1} " : Inport  PortDimensions=22
      mask Display: e = 0.06;c1 = [120 230 180]/255;c2 = ([120 230 180]+0)/(256+128);c3 = ([120 230 180]+128)/(256+128);patch([0 1 1 0],[0 0 1 1],c1);patch([0 1 1 1-e 1-e 0+e],[0 0 1 1-e 0+e 0+e],c2);patch([0 0 1 1-e 0+e 0+e],[0 1 1 1-e 1-e 0+e],c3);plot([0 1 1 0 0],[0 0 1 1 0]);
  Delays 1 : Subsystem
      mask Display: e = 0.06;c1 = [120 150 230]/255;c2 = ([120 150 230]+0)/383;c3 = ([120 150 230]+128)/383;patch([0 1 1 0],[0 0 1 1],c1);patch([0 1 1 1-e 1-e 0+e],[0 0 1 1-e 0+e 0+e],c2);patch([0 0 1 1-e 0+e 0+e],[0 1 1 1-e 1-e 0+e],c3);plot([0 1 1 0 0],[0 0 1 1 0]);disp('0');
  "LW{2,1}" : Subsystem
      mask Display: e = 0.06;c1 = [120 150 230]/255;c2 = ([120 150 230]+0)/383;c3 = ([120 150 230]+128)/383;patch([0 1 1 0],[0 0 1 1],c1);patch([0 1 1 1-e 1-e 0+e],[0 0 1 1-e 0+e 0+e],c2);patch([0 0 1 1-e 0+e 0+e],[0 1 1 1-e 1-e 0+e],c3);plot([0 1 1 0 0],[0 0 1 1 0]);disp('W');
  "b{2}" : Constant  Value=[1.5961384705337076095332804470672272145748138427734375;0.5017888253277231758175958020729012787342071533203125;-2.7030258154797675018699010252021253108978271484375;-2.733667787373037061371405798126943409442901611328125;1.9050591263444978107344240925158374011516571044921875;-1.837831736176462893439520485117100179195404052734375;0.58389981300689985932450554173556156456470489501953125;1.4419124619519931851385763366124592721462249755859375;-0.699327746355205448480774066410958766937255859375;-1.5325802103878973792205897552776150405406951904296875;-4.81942734529451310976355671300552785396575927734375;-0.476357098004361600995792969115427695214748382568359375]
      mask Display: e = 0.06;c1 = [120 150 230]/255;c2 = ([120 150 230]+0)/383;c3 = ([120 150 230]+128)/383;patch([0 1 1 0],[0 0 1 1],c1);patch([0 1 1 1-e 1-e 0+e],[0 0 1 1-e 0+e 0+e],c2);patch([0 0 1 1-e 0+e 0+e],[0 1 1 1-e 1-e 0+e],c3);plot([0 1 1 0 0],[0 0 1 1 0]);disp('b');
  netsum : Sum  Inputs=2  SaturateOnIntegerOverflow=on  InputSameDT=on  OutDataTypeStr=Inherit: Same as first input
      mask Display: e = 0.06;c1 = [120 150 230]/255;c2 = ([120 150 230]+0)/383;c3 = ([120 150 230]+128)/383;patch([0 1 1 0],[0 0 1 1],c1);patch([0 1 1 1-e 1-e 0+e],[0 0 1 1-e 0+e 0+e],c2);patch([0 0 1 1-e 0+e 0+e],[0 1 1 1-e 1-e 0+e],c3);plot([0 1 1 0 0],[0 0 1 1 0]);disp('+');
  tansig : neural/Transfer Functions/tansig
      settings: SourceProductName=Deep Learning Toolbox
  "a{2}" : Outport  InitialOutput=[0;0;0;0;0;0;0;0;0;0;0;0]
      mask Display: e = 0.06;c1 = [120 230 180]/255;c2 = ([120 230 180]+0)/(256+128);c3 = ([120 230 180]+128)/(256+128);patch([0 1 1 0],[0 0 1 1],c1);patch([0 1 1 1-e 1-e 0+e],[0 0 1 1-e 0+e 0+e],c2);patch([0 0 1 1-e 0+e 0+e],[0 1 1 1-e 1-e 0+e],c3);plot([0 1 1 0 0],[0 0 1 1 0]);
  wires:
  tansig/1 -> "a{2}"/1
  netsum/1 -> tansig/1
  "b{2}"/1 -> netsum/2
  "LW{2,1}"/1("lz{2,1}") -> netsum/1
  Delays 1/1("pd{2,1}") -> "LW{2,1}"/1("ad{2,1}")
  "a{1} "/1 -> Delays 1/1("p{2}")

== system motorai/PARAMETERS EXTIMATION HIL/Function Fitting Neural Network/Layer 3 ==
  "a{2} " : Inport  PortDimensions=12
      mask Display: e = 0.06;c1 = [120 230 180]/255;c2 = ([120 230 180]+0)/(256+128);c3 = ([120 230 180]+128)/(256+128);patch([0 1 1 0],[0 0 1 1],c1);patch([0 1 1 1-e 1-e 0+e],[0 0 1 1-e 0+e 0+e],c2);patch([0 0 1 1-e 0+e 0+e],[0 1 1 1-e 1-e 0+e],c3);plot([0 1 1 0 0],[0 0 1 1 0]);
  Delays 1 : Subsystem
      mask Display: e = 0.06;c1 = [120 150 230]/255;c2 = ([120 150 230]+0)/383;c3 = ([120 150 230]+128)/383;patch([0 1 1 0],[0 0 1 1],c1);patch([0 1 1 1-e 1-e 0+e],[0 0 1 1-e 0+e 0+e],c2);patch([0 0 1 1-e 0+e 0+e],[0 1 1 1-e 1-e 0+e],c3);plot([0 1 1 0 0],[0 0 1 1 0]);disp('0');
  "LW{3,2}" : Subsystem
      mask Display: e = 0.06;c1 = [120 150 230]/255;c2 = ([120 150 230]+0)/383;c3 = ([120 150 230]+128)/383;patch([0 1 1 0],[0 0 1 1],c1);patch([0 1 1 1-e 1-e 0+e],[0 0 1 1-e 0+e 0+e],c2);patch([0 0 1 1-e 0+e 0+e],[0 1 1 1-e 1-e 0+e],c3);plot([0 1 1 0 0],[0 0 1 1 0]);disp('W');
  "b{3}" : Constant  Value=[-2.90523246492434505938717848039232194423675537109375;-0.26630513715193393498026352972374297678470611572265625;-2.34697600092089242451720565441064536571502685546875;-4.03205637304003960963427743990905582904815673828125;0.9015766888685543545278733290615491569042205810546875]
      mask Display: e = 0.06;c1 = [120 150 230]/255;c2 = ([120 150 230]+0)/383;c3 = ([120 150 230]+128)/383;patch([0 1 1 0],[0 0 1 1],c1);patch([0 1 1 1-e 1-e 0+e],[0 0 1 1-e 0+e 0+e],c2);patch([0 0 1 1-e 0+e 0+e],[0 1 1 1-e 1-e 0+e],c3);plot([0 1 1 0 0],[0 0 1 1 0]);disp('b');
  netsum : Sum  Inputs=2  SaturateOnIntegerOverflow=on  InputSameDT=on  OutDataTypeStr=Inherit: Same as first input
      mask Display: e = 0.06;c1 = [120 150 230]/255;c2 = ([120 150 230]+0)/383;c3 = ([120 150 230]+128)/383;patch([0 1 1 0],[0 0 1 1],c1);patch([0 1 1 1-e 1-e 0+e],[0 0 1 1-e 0+e 0+e],c2);patch([0 0 1 1-e 0+e 0+e],[0 1 1 1-e 1-e 0+e],c3);plot([0 1 1 0 0],[0 0 1 1 0]);disp('+');
  purelin : neural/Transfer Functions/purelin
      settings: SourceProductName=Deep Learning Toolbox
  "a{3}" : Outport  InitialOutput=[0;0;0;0;0]
      mask Display: e = 0.06;c1 = [120 230 180]/255;c2 = ([120 230 180]+0)/(256+128);c3 = ([120 230 180]+128)/(256+128);patch([0 1 1 0],[0 0 1 1],c1);patch([0 1 1 1-e 1-e 0+e],[0 0 1 1-e 0+e 0+e],c2);patch([0 0 1 1-e 0+e 0+e],[0 1 1 1-e 1-e 0+e],c3);plot([0 1 1 0 0],[0 0 1 1 0]);
  wires:
  purelin/1 -> "a{3}"/1
  netsum/1 -> purelin/1
  "b{3}"/1 -> netsum/2
  "LW{3,2}"/1("lz{3,2}") -> netsum/1
  Delays 1/1("pd{3,2}") -> "LW{3,2}"/1("ad{3,2}")
  "a{2} "/1 -> Delays 1/1("p{3}")

== system motorai/PARAMETERS EXTIMATION HIL/Function Fitting Neural Network/Process Input 1 ==
  x : Inport  PortDimensions=100
      mask Display: e = 0.06;c1 = [120 230 180]/255;c2 = ([120 230 180]+0)/(256+128);c3 = ([120 230 180]+128)/(256+128);patch([0 1 1 0],[0 0 1 1],c1);patch([0 1 1 1-e 1-e 0+e],[0 0 1 1-e 0+e 0+e],c2);patch([0 0 1 1-e 0+e 0+e],[0 1 1 1-e 1-e 0+e],c3);plot([0 1 1 0 0],[0 0 1 1 0]);
  mapminmax : neural/Processing Functions/mapminmax  xmin=[-1.01752067813631819070963047125;-0.92595560019138756224776898307;-0.806514051643200668983979539917;-1.0958324073174869894842231588;-1.30056128835751749761584505904;-0.967267859388456829883295995387;-0.902840082408305266703507641068;-1.20787254563243817706563731917;-1.16585885786203569125518697547;-0.850823508957926244455904907227;-1.06870524100753638840899384377;-1.12465657319662204471910627035;-1.0516089277069688989740825491;-0.971783601593239954041791861528;-1.16269518113876446641086204181;-1.25029590123550082836345609394;-1.23511188346768396861818928301;-1.17612189100792674523177083756;-1.12019902279117622434512213658;-1.12300381316022890310080128984;-1.06251041206301310992898834229;-0.945709822363022478697303085937;-0.782251508182887134168481679808;-0.583762607623381613031199321995;-0.411909835320385553369959552583;-0.389627368284809427745329912796;-0.343436408716798702300820878008;-0.400070753509216336940568226055;-0.431752512062611559784386372485;-0.40041092548511397763988384213;-0.342764696985008610052858557538;-0.39812117701180488316126115933;-0.441749633088454607410255903233;-0.473911038586325938926080425517;-0.495023814014398599869792860773;-0.50564470567781538701268573277;-0.506449044715435170438411205396;-0.539211618118749846928494662279;-0.549883636365046779559406786575;-0.516911137957321464853066572687;-0.454988240589770998045793248821;-0.491452949874856492851193934257;-0.520645204372909065071439727035;-0.54279084783838205119366193685;-0.558166949034629045200972541352;-0.567095632632593771305096197466;-0.569937909213268589780909678666;-0.567087562958396906864777520241;-0.558965151016873162959086585033;0.00030642581492325147345459623871;0.000611989551039875687502012091556;0.000916631329361183833613624383219;0.00122035393165109608965002152559;0.00152316013128029476009217546562;0.00178477314709795244034029604308;0.00178477314709795244034029604308;0.00178477314709795244034029604308;0.00178477314709795244034029604308;0.00178477314709795244034029604308;0.00178477314709795244034029604308;0.00178477314709795244034029604308;0.00178477314709795244034029604308;0.00178477314709795244034029604308;0.00178477314709795244034029604308;0.00178477314709795244034029604308;0.00178477314709795244034029604308;0.00178477314709795244034029604308;0.00178477314709795244034029604308;0.00178477314709795244034029604308;0.00178477314709795244034029604308;0.00178477314709795244034029604308;0.00178477314709795244034029604308;0.00178477314709795244034029604308;0.00178477314709795244034029604308;0.00178477314709795244034029604308;0.00178477314709795244034029604308;0.00178477314709795244034029604308;0.00178477314709795244034029604308;0.00178477314709795244034029604308;0.00178477314709795244034029604308;0.00178477314709795244034029604308;0.00178477314709795244034029604308;0.00178477314709795244034029604308;0.00178477314709795244034029604308;0.00178477314709795244034029604308;0.00178477314709795244034029604308;0.00178477314709795244034029604308;0.00178477314709795244034029604308;0.00178477314709795244034029604308;0.00178477314709795244034029604308;0.00178477314709795244034029604308;0.00178477314709795244034029604308;0.00178477314709795244034029604308;0.00178477314709795244034029604308;0.00178477314709795244034029604308;0.00178477314709795244034029604308;0.00178477314709795244034029604308;0.00178477314709795244034029604308]  xmax=[9.80577218105379166956936387578;9.798753674793365675554923655;9.79709514650660651113867061213;9.79633539856964752345902525121;9.79598736897555433245088352123;9.7958279416280422680074480013;9.79575491025494926589090027846;9.79572145563414764524168276694;9.7957061305539063766900653718;9.79569911035523688269677222706;9.79569589450327526947148726322;9.79569442136777901453115191543;9.79569374654561464410562621197;9.7956934374192936587633084855;9.79569329581297765230374352541;9.79569323094515986838359822286;9.79569320123014719570164743345;9.79569318761812724005721975118;9.79569318138265821005461475579;9.80449275020298749439007224282;9.81433625111950469488419912523;9.8218125816725052601441348088;9.82749062326632127906123059802;9.83180265479931492222931410652;9.83507712112970189366478734883;9.8375635508336909396120972815;9.83945150120834988172191515332;9.8408849601222403435940577765;9.84197329274821797184813476633;9.84279956107103082274534244789;9.84342684599063133532581559848;9.84390305106861518424921086989;9.84426455222229535024780489039;9.84453897036720881885685230372;9.84474727759570988894211041043;9.84543846024130431260346085764;9.84850742187127536908519687131;9.85108819001237812074123212369;9.85325842379212879507122124778;9.85508342875237985936109907925;9.85661812198958919850610982394;9.85790868469140768581837619422;9.85899395179687410006863501621;9.85990658059712288263654045295;9.86067403344154236322083306732;9.8613194041204490503105262178;9.86186211279137481255929742474;9.86231849036030361332905158633;9.86270226990277443235299870139;231.921784288631727122265147045;243.027127918509023629667353816;258.392117274067402377113467082;276.519306233178610909817507491;303.056206938922969129635021091;308.13559860450573069101665169;301.787416620268800215853843838;295.033287653615445833565900102;298.320220726472769001702545211;319.582349957078463376092258841;339.171760464288922776177059859;354.781288895654768111853627488;366.871529461276111305778613314;375.939719527942770582740195096;382.481838726162777675199322402;386.966966914738918603688944131;389.821303905518448118527885526;391.419581950479596343939192593;392.081943700165936661505838856;392.074691334210513105063000694;391.613622157727093053836142644;390.86894342064920238044578582;389.971000215732601645868271589;389.016254082074851794459391385;388.073117691835022924351505935;387.187385506637212984060170129;386.387105187159647812222829089;385.686813842086678505438612774;385.091120980080347635521320626;384.597660171195570910640526563;384.199457497223761492932680994;383.886780030831005205982364714;383.648534545521840755100129172;383.473287694186865337542258203;383.349975855428851900796871632;383.268367204292587757663568482;383.219331451486539208417525515;383.194964959088167688605608419;383.1886111879377949662739411;383.194809074956822314561577514;383.209195236499283510056557134;383.228379987856953903246903792;383.249812113229268106806557626;383.271643106842645920551149175;383.292598184805456185131333768;383.311858663424175119871506467;383.328958224331131532380823046;383.343694046700875333044677973;383.356052690719252495910041034]  ymin=-1  ymax=1
      settings: SourceProductName=Deep Learning Toolbox
  removeconstantrows : neural/Processing Functions/removeconstantrows  inputSize=100  keep=[2 3 4 5 6 7 8 9 10 11 12 13 14 15 16 17 18 19 20 21 22 23 24 25 26 27 28 29 30 31 32 33 34 35 36 37 38 39 40 41 42 43 44 45 46 47 48 49 50 52 53 54 55 56 57 58 59 60 61 62 63 64 65 66 67 68 69 70 71 72 73 74 75 76 77 78 79 80 81 82 83 84 85 86 87 88 89 90 91 92 93 94 95 96 97 98 99 100]
      settings: SourceProductName=Deep Learning Toolbox  SourceProductBaseCode=NN
  p : Outport  PortDimensions=98
      mask Display: e = 0.06;c1 = [120 230 180]/255;c2 = ([120 230 180]+0)/(256+128);c3 = ([120 230 180]+128)/(256+128);patch([0 1 1 0],[0 0 1 1],c1);patch([0 1 1 1-e 1-e 0+e],[0 0 1 1-e 0+e 0+e],c2);patch([0 0 1 1-e 0+e 0+e],[0 1 1 1-e 1-e 0+e],c3);plot([0 1 1 0 0],[0 0 1 1 0]);
  wires:
  mapminmax/1 -> p/1
  removeconstantrows/1 -> mapminmax/1
  x/1 -> removeconstantrows/1

== system motorai/PARAMETERS EXTIMATION HIL/Function Fitting Neural Network/Process Output 1 ==
  a : Inport  PortDimensions=5
      mask Display: e = 0.06;c1 = [120 230 180]/255;c2 = ([120 230 180]+0)/(256+128);c3 = ([120 230 180]+128)/(256+128);patch([0 1 1 0],[0 0 1 1],c1);patch([0 1 1 1-e 1-e 0+e],[0 0 1 1-e 0+e 0+e],c2);patch([0 0 1 1-e 0+e 0+e],[0 1 1 1-e 1-e 0+e],c3);plot([0 1 1 0 0],[0 0 1 1 0]);
  mapminmax_reverse : neural/Processing Functions/mapminmax_reverse  xmin=[4.18330220693929888398088223767e-05;1.65640856421012117039026634302e-05;0.000361621201094397548558845301159;6.71152911148054087675518530887e-05;3.18777266080649823720705171581e-05]  xmax=[0.999976042031588185921009426238;0.99985988918983070838919502421;0.999955297151040700676105643652;0.999808456503088249789357178088;0.999863390300402943289270751848]  ymin=-1  ymax=1
      settings: SourceProductName=Deep Learning Toolbox
  y : Outport  PortDimensions=5
      mask Display: e = 0.06;c1 = [120 230 180]/255;c2 = ([120 230 180]+0)/(256+128);c3 = ([120 230 180]+128)/(256+128);patch([0 1 1 0],[0 0 1 1],c1);patch([0 1 1 1-e 1-e 0+e],[0 0 1 1-e 0+e 0+e],c2);patch([0 0 1 1-e 0+e 0+e],[0 1 1 1-e 1-e 0+e],c3);plot([0 1 1 0 0],[0 0 1 1 0]);
  wires:
  mapminmax_reverse/1 -> y/1
  a/1 -> mapminmax_reverse/1
